simulink subsystem "param_handler"  (R2023b)
settings: Solver=VariableStepAuto  StartTime=0.0  StopTime=10.0  RelTol=1e-3
model mask{rng_seed_f=0, sample_dim_f=0}
  mask prompts: rng_seed_f "rng seed"; sample_dim_f "sample dim"
values from neighbouring files (symbols this model uses):
  fs = f_resample    [inizio.m]    (also in load_preset_audio.m; resample_workspace.m)
settings Model: Creator=Edp  LastModifiedBy=giorg

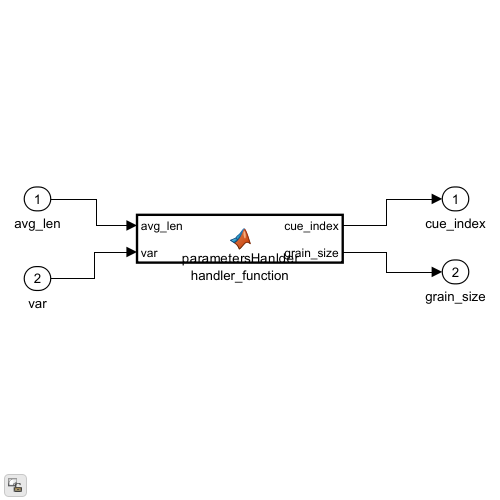
[thumbnail: Simulink's stored preview of the top-level diagram]
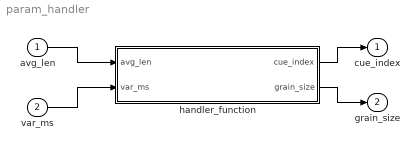
== system param_handler ==
  avg_len : Inport  OutDataTypeStr=double  PortDimensions=1  SampleTime=[0.01,0]
  var_ms : Inport  Port=2  OutDataTypeStr=double  PortDimensions=1
  handler_function : MATLAB Function  TreatAsAtomicUnit=on  mask{sample_dim_f=sample_dim_f, fs=fs, rng_seed_f=rng_seed_f}
      mask prompts: sample_dim_f "sample dimension"; fs "sampling frequency"; rng_seed_f "rng seed"
  cue_index : Outport  OutDataTypeStr=double  PortDimensions=1  SampleTime=[0.01,0]
  grain_size : Outport  Port=2  OutDataTypeStr=double  PortDimensions=1  SampleTime=[0.01,0]
  wires:
  var_ms/1 -> handler_function/2(var_ms)
  avg_len/1 -> handler_function/1(avg_len)
  handler_function/2(grain_size) -> grain_size/1
  handler_function/1(cue_index) -> cue_index/1

== matlab function param_handler/handler_function ==
  data: cue_index output; grain_size output; sample_dim_f parameter; avg_len input; var_ms input; rng_seed_f parameter; fs parameter
% INPUT: total input audio length (sample_dim_f), average computed length
% of the grain (avg_len), variation on the length of the grain in ms
% (var_ms), seeds of the random number generator (rng_seed_f), sampling
% frequency (fs)

% OUTPUT: starting point of the grain (cue_index), size of the grain (grain_size)

% This function takes in input the length of the grain, adds some
% variation, and outputs the grain size and the cue point of the randomly extracted grain
function [cue_index, grain_size] = parametersHanlder(sample_dim_f, avg_len, var_ms, rng_seed_f, fs)
   
    persistent random_start;
    if isempty(random_start)
        random_start = 1;
    end
    avg_len = min(sample_dim_f, avg_len);  % Grains can't be longer than the input audio file         
    rng(rng_seed_f);                       % Different seed for each handler 
    var = ceil((var_ms/1000)/(1/fs));  
    if random_start == 1                   % In the first iteration increase variance in any case 
        var = 40000;
        random_start = 0;
    end
    % If the maximum grain duration is too big avg_len must be equal to the input audio length
    % otherwise min_grain_size could be equal to max_grain_size
    min_grain_size = min(max(avg_len - var, 2048), sample_dim_f - 1);   % Lower bound for short grains 2048 samples
    max_grain_size = max(min(avg_len + var, sample_dim_f - 1), 1);
    grain_size = randi([floor(min_grain_size), floor(max_grain_size)]);
    cue_index = randi([1, sample_dim_f - floor(grain_size)]);
end
